simulink model "Model_ZN_FOPID"  (Simulink 9.2)
settings: Solver=VariableStepAuto  StartTime=0.0  StopTime=20  FixedStep=T_s  MaxStep=1e-3  RelTol=1e-3  EnableMultiTasking=on
values from neighbouring files (symbols this model uses):
  disturb_step_time = handles.disTime    [GUI_Comparison1.m]    (also in GUI_Comparison2.m; GUI_Main.m = str2double(get(handles.edit_disTime,   'string')); function_PI_lambdaD.m = 100; programEx6PILamD.m = 40)
  disturb_step_value = handles.disValue    [GUI_Comparison1.m]    (also in GUI_Comparison2.m; GUI_Main.m = str2double(get(handles.edit_disValue,  'string')); function_PI_lambdaD.m = 0.5; programEx6PILamD.m = 0.5)
  kdo = Kp*Td    [GUI_Comparison1.m]    (also in GUI_Comparison2.m; GUI_Main.m = handles.kdo; function_PI_lambdaD.m = fpp_kd(j); programEx6PILamD.m = 3.6466)
  kio = Kp/Ti    [GUI_Comparison1.m]    (also in GUI_Comparison2.m; GUI_Main.m = handles.kio; function_PI_lambdaD.m = fpp_ki(j); programEx6PILamD.m = 14.7942)
  kpo = Kp    [GUI_Comparison1.m]    (also in GUI_Comparison2.m; GUI_Main.m = handles.kpo; function_PI_lambdaD.m = fpp_kp(j); programEx6PILamD.m = 0.3835)
  L = handles.L    [GUI_Comparison1.m]    (also in GUI_Comparison2.m; GUI_Main.m; function_PI_lambdaD.m = delay; irid_fod.m = 200)
  step_value = handles.stepValue    [GUI_Comparison1.m]    (also in GUI_Comparison2.m; GUI_Main.m = str2double(get(handles.edit_stepValue, 'string')); programEx6PILamD.m = 1)
libraries: cstblocks x4, powerlib x1
settings Model: Creator=Li Chuang  LastModifiedBy=18764
settings SolverCC: AlgebraicLoopSolver=LineSearch
settings OptimizationCC: InitFltsAndDblsToZero=on
settings DebuggingCC: SaveWithParameterizedLinksMsg=none  SignalResolutionControl=TryResolveAllWithWarning  SolverPrmCheckMsg=warning  MultiTaskDSMMsg=warning  MultiTaskCondExecSysMsg=none  FcnCallInpInsideContextMsg=error  AllowSymbolicDim=off  StateNameClashWarn=none
settings GRTTargetCC: TargetFcnLib=ansi_tfl_tmw.mat  GeneratePreprocessorConditionals=Use local settings

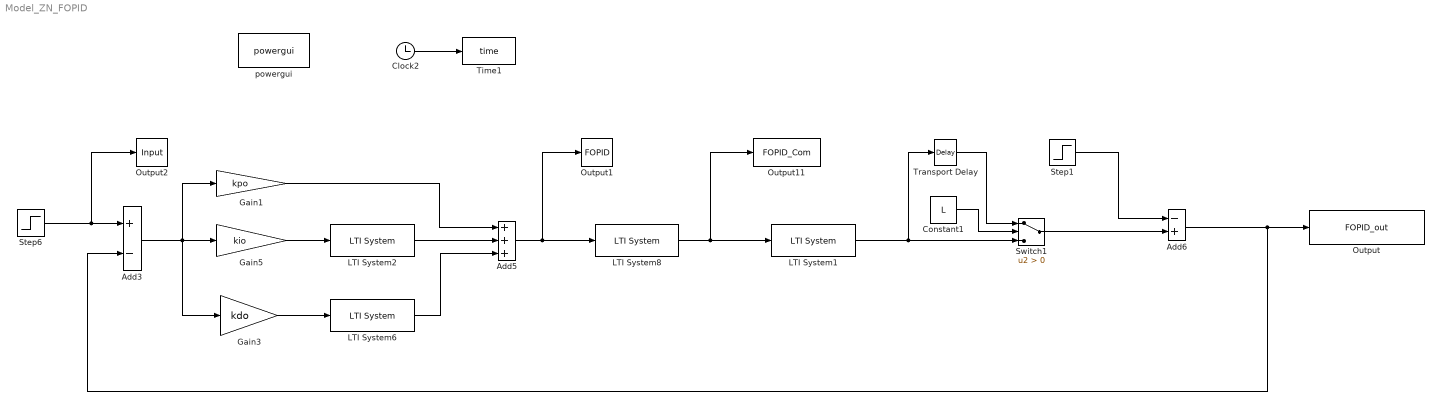
== system Model_ZN_FOPID ==
  Add3 : Sum  Inputs=+-  SaturateOnIntegerOverflow=on  OutDataTypeStr=Inherit: Same as first input
  Add5 : Sum  Inputs=+++  SaturateOnIntegerOverflow=on  OutDataTypeStr=Inherit: Same as first input
  Add6 : Sum  Inputs=-+  SaturateOnIntegerOverflow=on  OutDataTypeStr=Inherit: Same as first input
  Clock2 : Clock
      settings: Decimation=100
  Constant1 : Constant  Value=L
  Gain1 : Gain  Gain=kpo
  Gain3 : Gain  Gain=kdo
  Gain5 : Gain  Gain=kio
  LTI System1 : cstblocks/LTI System  sys=Gp  IC=[]
  LTI System2 : cstblocks/LTI System  sys=ifo  IC=[]
  LTI System6 : cstblocks/LTI System  sys=dfo  IC=[]
  LTI System8 : cstblocks/LTI System  sys=Ga  IC=[]
  Output : ToWorkspace  VariableName=FOPID_out  SampleTime=-1
  Output1 : ToWorkspace  VariableName=FOPID  SampleTime=-1
  Output11 : ToWorkspace  VariableName=FOPID_Com  SampleTime=-1
  Output2 : ToWorkspace  VariableName=Input  SampleTime=-1
  Step1 : Step  Time=disturb_step_time  After=disturb_step_value
  Step6 : Step  Time=0  After=step_value
  Switch1 : Switch  Criteria=u2 > Threshold
  Time1 : ToWorkspace  VariableName=time  SampleTime=-1
  Transport Delay : TransportDelay  DelayTime=L
  powergui : powerlib/powergui  Priority=1  SimulationMode=Continuous  SampleTime=50e-6  frequency=60  Iterations=50  frequencyindice=60  Pbase=100e6  ErrMax=1e-4  UnitsV=kV  UnitsW=MW  buscounter=0  FunctionMessages=off  echomessages=off  EnableUseOfTLC=off  CurrentSourceSwitches=off  DisableSnubberDevices=off  DisableRonSwitches=off  DisableVfSwitches=off  DisplayEquations=off  SolverType=Tustin/Backward Euler (TBE)  Interpol=off  ExternalGateDelay=off  methode=off  Ts=100  x0status=blocks  SPID=on  SwTol=0  HookPort=off  RestoreLinks=warning  ResistiveCurrentMeasurement=off  Frange=[0:2:500]  Ylog=off  Xlog=on  ShowGrid=off  save=off  variable=ZData  structure=0  ZoomFFT=off  StartTime=0.0  cycles=1  DisplayStyle=1  fundamental=60  FreqAxis=off  MaxFrequency=1000  frequencyindicesteady=1  RmsSteady=1  display=off
  wires:
  Add5/1 -> LTI System8/1, Output1/1
  Gain5/1 -> LTI System2/1
  Gain3/1 -> LTI System6/1
  LTI System6/1 -> Add5/3
  Add3/1 -> Gain1/1, Gain3/1, Gain5/1
  LTI System2/1 -> Add5/2
  Gain1/1 -> Add5/1
  Clock2/1 -> Time1/1
  Add6/1 -> Add3/2, Output/1
  Constant1/1 -> Switch1/2
  LTI System1/1 -> Switch1/3, Transport Delay/1
  Switch1/1 -> Add6/2
  Transport Delay/1 -> Switch1/1
  Step6/1 -> Output2/1, Add3/1
  Step1/1 -> Add6/1
  LTI System8/1 -> LTI System1/1, Output11/1
